simulink model "ABS"  (R2014a)
settings: Solver=ode45  StartTime=0.0  StopTime=100  RelTol=1e-3
values from neighbouring files (symbols this model uses):
  g = 9.81    [ABS script.m]
  I = 5    [ABS script.m]
  m = 80    [ABS script.m]
  r = 1.25    [ABS script.m]
  R = 1.25    [ABS script.m]
  v0 = 56    [ABS script.m]
  vo = 56    [ABS script.m]
settings Model: Creator=Preyash  LastModifiedBy=Preyash
settings DebuggingCC: SolverPrmCheckMsg=none

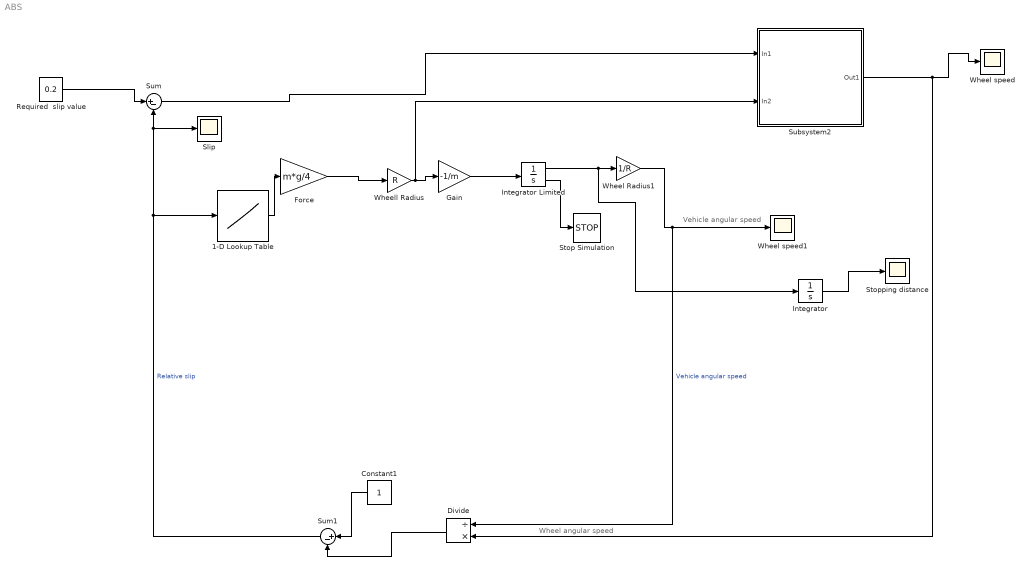
== system ABS ==
  note: Wheel angular speed
  note: Vehicle angular speed
  1-D Lookup Table : Lookup_n-D  NumberOfTableDimensions=1  BreakpointsForDimension1=[0,0.05,0.1,0.15,0.2,0.25,0.3,0.35,0.4,0.45,0.5,0.55,0.6,0.65,0.7,0.75,0.8,0.85,0.9,0.95,1]  Table=[0,0.4,0.8,0.97,1,0.98,0.96,0.94,0.92,0.9,0.88,0.855,0.83,0.81,0.79,0.77,0.75,0.73,0.72,0.71,0.7]  InternalRulePriority=Speed  RndMeth=Simplest  InputSameDT=on
  Constant1 : Constant
  Divide : Product  Inputs=/*
  Force : Gain  Gain=m*g/4
  Gain : Gain  Gain=-1/m
  Integrator : Integrator
  Integrator Limited : Integrator  InitialCondition=v0  LimitOutput=on  UpperSaturationLimit=1000  LowerSaturationLimit=0  ShowSaturationPort=on
  "Required  slip value " : Constant  Value=0.2
  "Slip " : Scope
      settings: SaveName=ScopeData3
  Stop Simulation : Stop
  Stopping distance : Scope
      settings: SaveName=ScopeData2
  Subsystem2 : Subsystem
  Sum : Sum  Inputs=|+-
  Sum1 : Sum  Inputs=|+-
  Wheel Radius1 : Gain  Gain=1/R
  Wheel speed : Scope
  Wheel speed1 : Scope
  Wheell Radius : Gain  Gain=R
  wires:
  "Required  slip value "/1 -> Sum/1
  Force/1 -> Wheell Radius/1
  Gain/1 -> Integrator Limited/1
  Integrator Limited/2 -> Stop Simulation/1
  Integrator Limited/1 -> Integrator/1, Wheel Radius1/1
  Wheell Radius/1 -> Subsystem2/2(In2), Gain/1
  Sum/1 -> Subsystem2/1(In1)
  Integrator/1 -> Stopping distance/1
  Constant1/1 -> Sum1/1
  Subsystem2/1(Out1) -> Divide/2, Wheel speed/1
  Divide/1 -> Sum1/2
  Wheel Radius1/1 -> Divide/1, Wheel speed1/1  "Vehicle angular speed"
  Sum1/1 -> 1-D Lookup Table/1, "Slip "/1, Sum/2  "Relative slip"
  1-D Lookup Table/1 -> Force/1

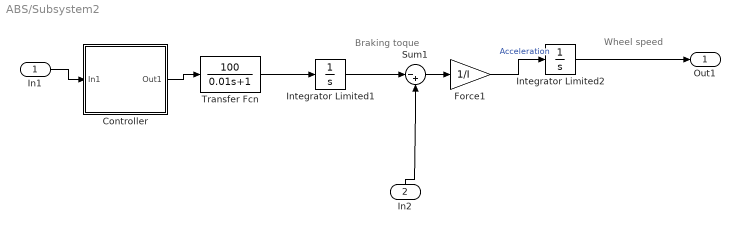
== system ABS/Subsystem2 ==
  note: Wheel speed
  note: Braking toque
  In1 : Inport
  In2 : Inport  Port=2
  "Controller " : Subsystem
  Force1 : Gain  Gain=1/I
  Integrator Limited1 : Integrator  LimitOutput=on  UpperSaturationLimit=1000  LowerSaturationLimit=0
  Integrator Limited2 : Integrator  InitialCondition=vo/r  LimitOutput=on  UpperSaturationLimit=1000  LowerSaturationLimit=0
  Sum1 : Sum  Inputs=|-+
  Transfer Fcn : TransferFcn  Numerator=[100]  Denominator=[0.01 1]
  Out1 : Outport
  wires:
  Sum1/1 -> Force1/1
  Integrator Limited1/1 -> Sum1/1
  In1/1 -> "Controller "/1(In1)
  "Controller "/1(Out1) -> Transfer Fcn/1
  Force1/1 -> Integrator Limited2/1  "Acceleration"
  In2/1 -> Sum1/2
  Transfer Fcn/1 -> Integrator Limited1/1
  Integrator Limited2/1 -> Out1/1

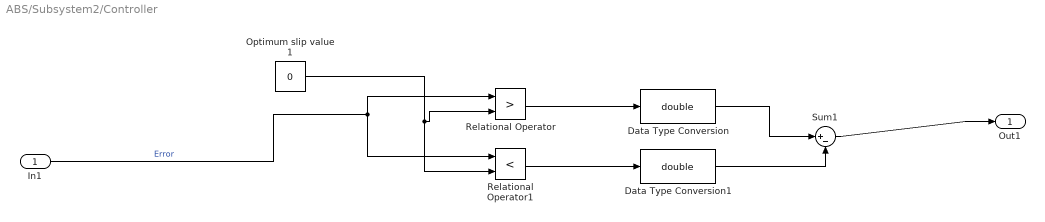
== system ABS/Subsystem2/Controller  ==
  In1 : Inport
  Data Type Conversion : DataTypeConversion  OutDataTypeStr=double  RndMeth=Zero
  Data Type Conversion1 : DataTypeConversion  OutDataTypeStr=double
  Optimum slip value 1 : Constant  Value=0
  Relational Operator : RelationalOperator  Operator=>  OutDataTypeStr=boolean
  Relational Operator1 : RelationalOperator  Operator=<  OutDataTypeStr=boolean
  Sum1 : Sum  Inputs=|+-
  Out1 : Outport
  wires:
  In1/1 -> Relational Operator/1, Relational Operator1/1  "Error"
  Relational Operator1/1 -> Data Type Conversion1/1
  Sum1/1 -> Out1/1
  Data Type Conversion1/1 -> Sum1/2
  Data Type Conversion/1 -> Sum1/1
  Relational Operator/1 -> Data Type Conversion/1
  Optimum slip value 1/1 -> Relational Operator/2, Relational Operator1/2
